simulink model "LinearBPS_inTransferFunction"  (R2023b)
settings: Solver=VariableStepAuto  StartTime=0.0  StopTime=10.0  RelTol=1e-3
settings Model: Creator=msdbg  LastModifiedBy=msdbg

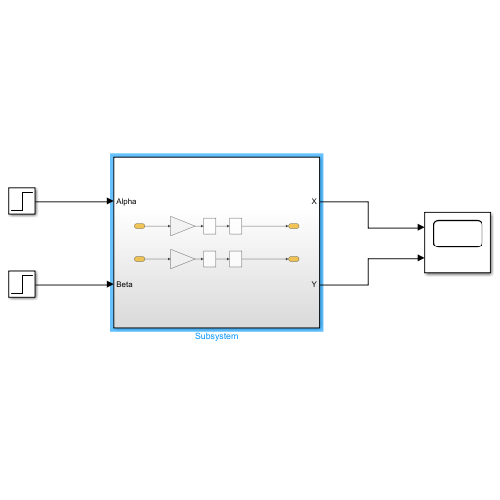
[thumbnail: Simulink's stored preview of the top-level diagram]
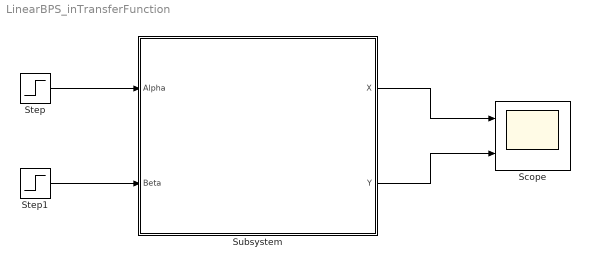
== system LinearBPS_inTransferFunction ==
  Scope : Scope  NumInputPorts=2
  Step : Step  After=3.14/10  SampleTime=0
  Step1 : Step  After=3.14/10  SampleTime=0
  Subsystem : Subsystem
  wires:
  Subsystem/1(X) -> Scope/1
  Subsystem/2(Y) -> Scope/2
  Step/1 -> Subsystem/1(Alpha)
  Step1/1 -> Subsystem/2(Beta)

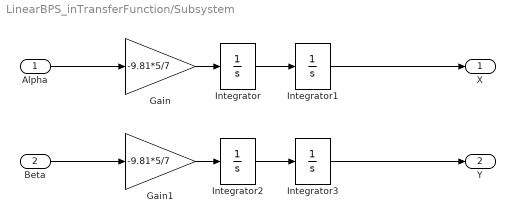
== system LinearBPS_inTransferFunction/Subsystem ==
  Alpha : Inport
  Beta : Inport  Port=2
  Gain : Gain  Gain=-9.81*5/7
  Gain1 : Gain  Gain=-9.81*5/7
  Integrator{,1..3} (4 alike) : Integrator
  X : Outport
  Y : Outport  Port=2
  wires:
  Gain1/1 -> Integrator2/1
  Alpha/1 -> Gain/1
  Gain/1 -> Integrator/1
  Beta/1 -> Gain1/1
  Integrator3/1 -> Y/1
  Integrator2/1 -> Integrator3/1
  Integrator/1 -> Integrator1/1
  Integrator1/1 -> X/1
